simulink model "LW_ctrl"  (R2024b)
settings: Solver=ode4  StartTime=0.0  StopTime=SIM_TIME  FixedStep=0.001  RelTol=1e-3  EnableMultiTasking=on
StartFcn:
  | %timestart = cputime;
StopFcn:
  | %dt = cputime - timestart
undefined symbols (not defined in the file or in its folder): AttCtrl_cycle, ControlMode, DEG2RAD, Earth, FlightMode, LW_ACRO_P_MAX, LW_ACRO_R_MAX, LW_ACRO_Y_MAX, LW_AERO_C0, LW_AERO_C1, LW_AERO_Y0, LW_ANGLE, LW_DMZ0, LW_DMZ_MIN, LW_LAT_CIRCLE, LW_MAN_PITCH_MAX, LW_MAN_ROLL_MAX, LW_MASS, LW_OB_CIRCLE_R, LW_OB_CIRCLE_V, LW_OB_CIRCLE_W, LW_OB_TYPE, LW_REX_YAW, LW_SERVOL_MAX, LW_SERVOR_MAX, LW_THR_HOVER, LW_WZ_MAX, LW_X_ACCEL_MAX, LW_X_ACCEL_MIN, LW_X_FF, LW_X_JERK_MAX, LW_X_P, LW_X_VEL_MAX, LW_Y_ACCEL_MAX, LW_Y_ACCEL_MIN, LW_Y_FF, LW_Y_JERK_MAX, LW_Y_P, LW_Y_VEL_MAX, LW_YAW_KAD, LW_YAW_KAP, LW_Z_ACCEL_LOW, LW_Z_ACCEL_UP, LW_Z_FF, LW_Z_JERK_MAX, LW_Z_P, LW_Z_VEL_MAX_UP, Map_xoffset, Map_yoffset, Map_zoffset, MAX_wdotx, MAX_wdoty, MAX_wdotz, Mixer_cycle, ModelParam_AccelMax, ModelParam_DelayAtt, ModelParam_DelayOmega, ModelParam_DelayPos, ModelParam_envAltitude, ModelParam_envGravityAcc ... (+57)
libraries: pixhawk_slib_uORB_RW x15, simulink x6, slpidlib x6, dspstat3 x5, aerolibnav x4, aerolibtransform2 x3, pixhawk_slib_sensors_actuators x2, etargetslib x2, pixhawk_slib_rfly x1, aerolibatmos2 x1, slrealtimeiplib x1, SignalEditorBlockLib x1
(part 6 of 6)

== matlab function LW_ctrl/navigator/navigator_manual/vy_deadzone ==
  data: u input; y output; LW_Y_VEL_DZ parameter
function y = fcn(u, LW_Y_VEL_DZ)
%Function description:
%  set a dead zone with a dead zone size of ±deadZone.
RCMin = single(-1);
RCMax = single(1);
RCMid = ((RCMin + RCMax)/2);
deadZone = LW_Y_VEL_DZ;
k = 1/(RCMax - RCMid - deadZone);

%dead zone
if(u > RCMid + deadZone)
    y = single((u-RCMid - deadZone)*k);
elseif(u < RCMid - deadZone)
    y = single((u - RCMid + deadZone)*k);
else
    y = single(0);
end
end

== matlab function LW_ctrl/navigator/navigator_manual/vz_deadzone ==
  data: u input; y output; LW_Z_VEL_DZ parameter
function y = fcn(u, LW_Z_VEL_DZ)
%Function description:
%  set a dead zone with a dead zone size of ±deadZone.
% u:0-1
u = u*2 - 1; % -1~1
RCMin = single(-1);
RCMax = single(1);
RCMid = ((RCMin + RCMax)/2);
deadZone = LW_Z_VEL_DZ;
k = 1/(RCMax - RCMid - deadZone);

%dead zone
if(u > RCMid + deadZone)
    y = single((u-RCMid - deadZone)*k);
elseif(u < RCMid - deadZone)
    y = single((u - RCMid + deadZone)*k);
else
    y = single(0);
end
end

== matlab function LW_ctrl/rc_receive/manual_ctrl_in/Sim/Simulate ref/commandMapping/command2pwm/stabilized/roll_deadzone_inv ==
  data: u input; y output; LW_MAN_ROLL_DZ parameter
function y = fcn(u, LW_MAN_ROLL_DZ)
%Function description:
%  set a dead zone with a dead zone size of ±deadZone.
RCMin = single(-1);
RCMax = single(1);
RCMid = ((RCMin + RCMax)/2);
deadZone = LW_MAN_ROLL_DZ;
k = 1/(RCMax - RCMid - deadZone);

%dead zone
if(u > RCMid + deadZone)
    y = single(u/k + RCMid + deadZone);
elseif(u < RCMid - deadZone)
     y = single(u/k + RCMid - deadZone);
else
    y = single(0);
end
end

== matlab function LW_ctrl/rc_receive/manual_ctrl_in/Sim/Simulate ref/commandMapping/command2pwm/stabilized/pitch_deadzone_inv ==
  data: u input; y output; LW_MAN_PITCH_DZ parameter
function y = fcn(u, LW_MAN_PITCH_DZ)
%Function description:
%  set a dead zone with a dead zone size of ±deadZone.
RCMin = single(-1);
RCMax = single(1);
RCMid = ((RCMin + RCMax)/2);
deadZone = LW_MAN_PITCH_DZ;
k = 1/(RCMax - RCMid - deadZone);

%dead zone
if(u > RCMid + deadZone)
    y = single(u/k + RCMid + deadZone);
elseif(u < RCMid - deadZone)
     y = single(u/k + RCMid - deadZone);
else
    y = single(0);
end
end

== matlab function LW_ctrl/rc_receive/manual_ctrl_in/Sim/Simulate ref/commandMapping/command2pwm/stabilized/yawrare_deadzone_inv ==
  data: u input; y output; LW_MAN_WZ_DZ parameter
function y = fcn(u, LW_MAN_WZ_DZ)
%Function description:
%  set a dead zone with a dead zone size of ±deadZone.
RCMin = single(-1);
RCMax = single(1);
RCMid = ((RCMin + RCMax)/2);
deadZone = LW_MAN_WZ_DZ;
k = 1/(RCMax - RCMid - deadZone);

%dead zone
if(u > RCMid + deadZone)
    y = single(u/k + RCMid + deadZone);
elseif(u < RCMid - deadZone)
     y = single(u/k + RCMid - deadZone);
else
    y = single(0);
end
end

== matlab function LW_ctrl/rc_receive/manual_ctrl_in/Sim/Simulate ref/commandMapping/command2pwm/altitude/pitch_deadzone_inv ==
  data: u input; y output; LW_MAN_PITCH_DZ parameter
function y = fcn(u, LW_MAN_PITCH_DZ)
%Function description:
%  set a dead zone with a dead zone size of ±deadZone.
RCMin = single(-1);
RCMax = single(1);
RCMid = ((RCMin + RCMax)/2);
deadZone = LW_MAN_PITCH_DZ;
k = 1/(RCMax - RCMid - deadZone);

%dead zone
if(u > RCMid + deadZone)
    y = single(u/k + RCMid + deadZone);
elseif(u < RCMid - deadZone)
     y = single(u/k + RCMid - deadZone);
else
    y = single(0);
end
end

== matlab function LW_ctrl/rc_receive/manual_ctrl_in/Sim/Simulate ref/commandMapping/command2pwm/altitude/roll_deadzone_inv ==
  data: u input; y output; LW_MAN_ROLL_DZ parameter
function y = fcn(u, LW_MAN_ROLL_DZ)
%Function description:
%  set a dead zone with a dead zone size of ±deadZone.
RCMin = single(-1);
RCMax = single(1);
RCMid = ((RCMin + RCMax)/2);
deadZone = LW_MAN_ROLL_DZ;
k = 1/(RCMax - RCMid - deadZone);

%dead zone
if(u > RCMid + deadZone)
    y = single(u/k + RCMid + deadZone);
elseif(u < RCMid - deadZone)
     y = single(u/k + RCMid - deadZone);
else
    y = single(0);
end
end

== matlab function LW_ctrl/rc_receive/manual_ctrl_in/Sim/Simulate ref/commandMapping/command2pwm/acro/wz_deadzone_inv ==
  data: u input; y output; LW_MAN_WZ_DZ parameter
function y = fcn(u, LW_MAN_WZ_DZ)
%Function description:
%  set a dead zone with a dead zone size of ±deadZone.
RCMin = single(-1);
RCMax = single(1);
RCMid = ((RCMin + RCMax)/2);
deadZone = LW_MAN_WZ_DZ;
k = 1/(RCMax - RCMid - deadZone);

%dead zone
if(u > RCMid + deadZone)
    y = single(u/k + RCMid + deadZone);
elseif(u < RCMid - deadZone)
     y = single(u/k + RCMid - deadZone);
else
    y = single(0);
end
end

== matlab function LW_ctrl/rc_receive/manual_ctrl_in/Sim/Simulate ref/commandMapping/command2pwm/acro/wx_deadzone_inv ==
  data: u input; y output; LW_MAN_WX_DZ parameter
function y = fcn(u, LW_MAN_WX_DZ)
%Function description:
%  set a dead zone with a dead zone size of ±deadZone.
RCMin = single(-1);
RCMax = single(1);
RCMid = ((RCMin + RCMax)/2);
deadZone = LW_MAN_WX_DZ;
k = 1/(RCMax - RCMid - deadZone);

%dead zone
if(u > RCMid + deadZone)
    y = single(u/k + RCMid + deadZone);
elseif(u < RCMid - deadZone)
     y = single(u/k + RCMid - deadZone);
else
    y = single(0);
end
end

== matlab function LW_ctrl/rc_receive/manual_ctrl_in/Sim/Simulate ref/commandMapping/command2pwm/acro/wy_deadzone_inv ==
  data: u input; y output; LW_MAN_WY_DZ parameter
function y = fcn(u, LW_MAN_WY_DZ)
%Function description:
%  set a dead zone with a dead zone size of ±deadZone.
RCMin = single(-1);
RCMax = single(1);
RCMid = ((RCMin + RCMax)/2);
deadZone = LW_MAN_WY_DZ;
k = 1/(RCMax - RCMid - deadZone);

%dead zone
if(u > RCMid + deadZone)
    y = single(u/k + RCMid + deadZone);
elseif(u < RCMid - deadZone)
     y = single(u/k + RCMid - deadZone);
else
    y = single(0);
end
end

== matlab function LW_ctrl/rc_receive/manual_ctrl_in/Sim/Simulate ref/commandMapping/command2pwm/position/wz_deadzone_inv ==
  data: u input; y output; LW_MAN_WZ_DZ parameter
function y = fcn(u, LW_MAN_WZ_DZ)
%Function description:
%  set a dead zone with a dead zone size of ±deadZone.
RCMin = single(-1);
RCMax = single(1);
RCMid = ((RCMin + RCMax)/2);
deadZone = LW_MAN_WZ_DZ;
k = 1/(RCMax - RCMid - deadZone);

%dead zone
if(u > RCMid + deadZone)
    y = single(u/k + RCMid + deadZone);
elseif(u < RCMid - deadZone)
     y = single(u/k + RCMid - deadZone);
else
    y = single(0);
end
end

== matlab function LW_ctrl/rc_receive/manual_ctrl_in/Sim/Simulate ref/commandMapping/command2pwm/position/vz_deadzone_inv ==
  data: u input; y output; LW_Z_VEL_DZ parameter
function y = fcn(u, LW_Z_VEL_DZ)
%Function description:
%  set a dead zone with a dead zone size of ±deadZone.
RCMin = single(-1);
RCMax = single(1);
RCMid = ((RCMin + RCMax)/2);
deadZone = LW_Z_VEL_DZ;
k = 1/(RCMax - RCMid - deadZone);

%dead zone
if(u > RCMid + deadZone)
    y = single(u/k + RCMid + deadZone);
elseif(u < RCMid - deadZone)
     y = single(u/k + RCMid - deadZone);
else
    y = single(0);
end

y = (y+1)*0.5;
end

== matlab function LW_ctrl/rc_receive/manual_ctrl_in/Sim/Simulate ref/commandMapping/command2pwm/position/vy_deadzone_inv ==
  data: u input; y output; LW_Y_VEL_DZ parameter
function y = fcn(u, LW_Y_VEL_DZ)
%Function description:
%  set a dead zone with a dead zone size of ±deadZone.
RCMin = single(-1);
RCMax = single(1);
RCMid = ((RCMin + RCMax)/2);
deadZone = LW_Y_VEL_DZ;
k = 1/(RCMax - RCMid - deadZone);

%dead zone
if(u > RCMid + deadZone)
    y = single(u/k + RCMid + deadZone);
elseif(u < RCMid - deadZone)
     y = single(u/k + RCMid - deadZone);
else
    y = single(0);
end
end

== matlab function LW_ctrl/rc_receive/manual_ctrl_in/Sim/Simulate ref/commandMapping/command2pwm/position/vx_deadzone_inv ==
  data: u input; y output; LW_X_VEL_DZ parameter
function y = fcn(u, LW_X_VEL_DZ)
%Function description:
%  set a dead zone with a dead zone size of ±deadZone.
RCMin = single(-1);
RCMax = single(1);
RCMid = ((RCMin + RCMax)/2);
deadZone = LW_X_VEL_DZ;
k = 1/(RCMax - RCMid - deadZone);

%dead zone
if(u > RCMid + deadZone)
    y = single(u/k + RCMid + deadZone);
elseif(u < RCMid - deadZone)
     y = single(u/k + RCMid - deadZone);
else
    y = single(0);
end
end

== matlab function LW_ctrl/rc_receive/manual_ctrl_in/Sim/Simulate ref/commandMapping/command2pwm/altitude/vz_deadzone_inv ==
  data: u input; y output; LW_Z_VEL_DZ parameter
function y = fcn(u, LW_Z_VEL_DZ)
%Function description:
%  set a dead zone with a dead zone size of ±deadZone.
RCMin = single(-1);
RCMax = single(1);
RCMid = ((RCMin + RCMax)/2);
deadZone = LW_Z_VEL_DZ;
k = 1/(RCMax - RCMid - deadZone);

%dead zone
if(u > RCMid + deadZone)
    y = single(u/k + RCMid + deadZone);
elseif(u < RCMid - deadZone)
     y = single(u/k + RCMid - deadZone);
else
    y = single(0);
end

y = (y+1)*0.5;
end

== matlab function LW_ctrl/rc_receive/manual_ctrl_in/Sim/Simulate ref/commandMapping/command2pwm/altitude/wz_deadzone_inv ==
  data: u input; y output; LW_MAN_WZ_DZ parameter
function y = fcn(u, LW_MAN_WZ_DZ)
%Function description:
%  set a dead zone with a dead zone size of ±deadZone.
RCMin = single(-1);
RCMax = single(1);
RCMid = ((RCMin + RCMax)/2);
deadZone = LW_MAN_WZ_DZ;
k = 1/(RCMax - RCMid - deadZone);

%dead zone
if(u > RCMid + deadZone)
    y = single(u/k + RCMid + deadZone);
elseif(u < RCMid - deadZone)
     y = single(u/k + RCMid - deadZone);
else
    y = single(0);
end
end

== matlab function LW_ctrl/states_update/vehicle_local_position/Sim/getIncid ==
  data: q input; incid output; LW_ANGLE parameter
function incid = fcn(q, LW_ANGLE)

if notInfNan(q)
    euler = my_quat2eul(q);
else
    euler = single([0;0;0]);
end
theta = euler(2);
alpha = theta + LW_ANGLE*pi/180;
beta = single(0);
incid = [alpha; beta];

== matlab function LW_ctrl/navigator/navigator_manual/Lowpass ==
  data: data_in input; data_in output; LW_VEL_DT parameter
function data_in = fcn(data_in, LW_VEL_DT)
persistent data_last
if isempty(data_last)
    data_last = data_in;
end
if isInfNan(data_last)
    data_last = single(0);
end

data_in = data_last + LW_VEL_DT*(data_in - data_last);
data_last = data_in;

== matlab function LW_ctrl/navigator/navigator_manual/Lowpass1 ==
  data: data_in input; data_in output; LW_VEL_DT parameter
function data_in = fcn(data_in, LW_VEL_DT)
persistent data_last
if isempty(data_last)
    data_last = data_in;
end
if isInfNan(data_last)
    data_last = single(0);
end

data_in = data_last + LW_VEL_DT*(data_in - data_last);
data_last = data_in;

== matlab function LW_ctrl/Output/OutputSelect/Sim/Lifting Body Airframe/Estimator/Sensor Model/GPS/GenCogVel ==
  data: v output; u input; cot output
function [v,cot] = Ang360(u)
v=norm(u(1:2));

if v < 1
    cot = 0;
else
    cot=atan2d(u(2),u(1));
end
 
if cot<0
    cot=cot+360;
end

== matlab function LW_ctrl/navigator/logger/Sim/quat2eul ==
  data: q input; euler output
function euler = fcn(q)
q = single(q);
euler = my_quat2eul(q,'ZYX');

== matlab function LW_ctrl/Output/OutputSelect/Sim/Lifting Body Airframe/Estimator/Sensor Model/Magnetometer Hub/MATLAB Function ==
  data: DCM input; mag_e input; b_m input; n_m input; Mag_means output; K_m input
function Mag_means = fcn(DCM, mag_e, b_m, n_m, K_m)
 
Mag_means = K_m*DCM*mag_e + b_m + n_m;

== matlab function LW_ctrl/Output/OutputSelect/Sim/Lifting Body Airframe/Estimator/Sensor Model/Magnetometer Hub/MATLAB Function1 ==
  data: DCM input; mag_e input; b_m input; n_m input; Mag_means output; K_m input
function Mag_means = fcn(DCM, mag_e, b_m, n_m, K_m)
 
Mag_means = K_m*DCM*mag_e + b_m + n_m;

== matlab function LW_ctrl/navigator/navigator_manual/nan_inf0 ==
  data: u input; y output
function y = fcn(u)

for i = 1:length(u)
    if isnan(u(i)) || isinf(u(i))
        u(i) = single(0);
    end
end
y = u;

== matlab function LW_ctrl/navigator/navigator_manual/nan_inf1 ==
  data: u input; y output
function y = fcn(u)

for i = 1:length(u)
    if isnan(u(i)) || isinf(u(i))
        u(i) = single(0);
    end
end
y = u;

== matlab function LW_ctrl/navigator/navigator_manual/nan_inf2 ==
  data: u input; y output
function y = fcn(u)

for i = 1:length(u)
    if isnan(u(i)) || isinf(u(i))
        u(i) = single(0);
    end
end
y = u;

== matlab function LW_ctrl/navigator/navigator_manual/nan_inf3 ==
  data: u input; y output
function y = fcn(u)

for i = 1:length(u)
    if isnan(u(i)) || isinf(u(i))
        u(i) = single(0);
    end
end
y = u;

== matlab function LW_ctrl/navigator/navigator_manual/nan_inf4 ==
  data: u input; y output
function y = fcn(u)

for i = 1:length(u)
    if isnan(u(i)) || isinf(u(i))
        u(i) = single(0);
    end
end
y = u;

== matlab function LW_ctrl/navigator/navigator_manual/nan_inf5 ==
  data: u input; y output
function y = fcn(u)

for i = 1:length(u)
    if isnan(u(i)) || isinf(u(i))
        u(i) = single(0);
    end
end
y = u;

== matlab function LW_ctrl/navigator/navigator_manual/nan_inf6 ==
  data: u input; y output
function y = fcn(u)

for i = 1:length(u)
    if isnan(u(i)) || isinf(u(i))
        u(i) = single(0);
    end
end
y = u;

== matlab function LW_ctrl/navigator/navigator_manual/nan_inf7 ==
  data: u input; y output
function y = fcn(u)

for i = 1:length(u)
    if isnan(u(i)) || isinf(u(i))
        u(i) = single(0);
    end
end
y = u;

== matlab function LW_ctrl/navigator/navigator_manual/nan_inf8 ==
  data: u input; y output
function y = fcn(u)

for i = 1:length(u)
    if isnan(u(i)) || isinf(u(i))
        u(i) = single(0);
    end
end
y = u;

== matlab function LW_ctrl/rc_receive/manual_ctrl_in/Sim/Simulate ref/commandMapping/MATLAB Function ==
  data: flight_mode input; AU8 output
function AU8 = fcn(flight_mode)
if flight_mode == FlightMode.PILOT
    AU8 = 1000;
elseif flight_mode == FlightMode.AUTO
    AU8 = 1500;
else
    %offboard
    AU8 = 2000;
end

== matlab function LW_ctrl/state_machine/MATLAB Function4 ==
  data: ctrl_mode output; ch5 input; ch7 input; ch8 input; flight_mode output; RC_Lost input; armed input
function [ctrl_mode, flight_mode]  = fcn(ch5, ch7, ch8, RC_Lost, armed)
%Function description:
%  Map the remote control CH5 channel to control mode
%input:
%  ch5: Remote control CH5 channel input
%  control_mode: Custom control mode
%  0: stablelize mode；1: height control mode; 2: position control mode
%  4: attitude rate mode
%  the remote control CH8 channel change the flight mode
%input:
%  ch8: Remote control CH8 channel input

if ch5 < 1400
    ctrl_mode = ControlMode.STABILIZED;
    if ch7 >1300 && ch7 < 1600
        %ctrl_mode = ControlMode.ACRO;
    elseif ch7 >= 1600
        ctrl_mode = ControlMode.MANUAL;
    end
elseif ch5 < 1600
    ctrl_mode = ControlMode.ALTITUDE;
else
    ctrl_mode = ControlMode.POSITION;
end
if ch8 < 1400
    flight_mode = FlightMode.PILOT;
% elseif ch8 < 1600
%     flight_mode = FlightMode.AUTO;
%     ctrl_mode = ControlMode.MISSION;
else
    flight_mode = FlightMode.OFFBOARD;
end

if RC_Lost > 0.5
%     flight_mode = FlightMode.AUTO;
%     ctrl_mode = ControlMode.LOITER;
end

% if armed > 0.5 && ch8 > 1500
%     flight_mode = FlightMode.OFFBOARD;
% end

== matlab function LW_ctrl/Output/OutputSelect/Sim/Lifting Body Airframe/Estimator/nan_inf ==
  data: u input; y output
function y = fcn(u)

for i = 1:length(u)
    if isnan(u(i)) || isinf(u(i))
        u(i) = 0;
    end
end
y = u;

== matlab function LW_ctrl/Output/OutputSelect/Sim/Lifting Body Airframe/Estimator/nan_inf1 ==
  data: u input; y output
function y = fcn(u)

for i = 1:length(u)
    if isnan(u(i)) || isinf(u(i))
        u(i) = 0;
    end
end
y = u;

== matlab function LW_ctrl/navigator/navigator_manual/nan_inf10 ==
  data: u input; y output
function y = fcn(u)

for i = 1:length(u)
    if isnan(u(i)) || isinf(u(i))
        u(i) = single(0);
    end
end
y = u;

== matlab function LW_ctrl/Output/OutputSelect/Sim/Lifting Body Airframe/Estimator/nan_inf2 ==
  data: u input; y output
function y = fcn(u)

for i = 1:length(u)
    if isnan(u(i)) || isinf(u(i))
        u(i) = 0;
    end
end
y = u;

== matlab function LW_ctrl/Output/OutputSelect/Sim/Lifting Body Airframe/Estimator/nan_inf3 ==
  data: u input; y output
function y = fcn(u)

for i = 1:length(u)
    if isnan(u(i)) || isinf(u(i))
        u(i) = 0;
    end
end
y = u;

== matlab function LW_ctrl/Output/OutputSelect/Sim/Lifting Body Airframe/Estimator/nan_inf4 ==
  data: u input; y output
function y = fcn(u)

for i = 1:length(u)
    if isnan(u(i)) || isinf(u(i))
        u(i) = 0;
    end
end
y = u;

== matlab function LW_ctrl/Output/OutputSelect/Sim/Lifting Body Airframe/Estimator/nan_inf5 ==
  data: u input; y output
function y = fcn(u)

for i = 1:length(u)
    if isnan(u(i)) || isinf(u(i))
        u(i) = 0;
    end
end
y = u;

== matlab function LW_ctrl/Output/OutputSelect/Sim/Lifting Body Airframe/Estimator/nan_inf6 ==
  data: u input; y output
function y = fcn(u)

for i = 1:length(u)
    if isnan(u(i)) || isinf(u(i))
        u(i) = 15;
    end
end
y = u;

== matlab function LW_ctrl/Output/OutputSelect/Sim/Lifting Body Airframe/Estimator/nan_inf_q ==
  data: u input; y output
function y = fcn(u)

for i = 1:length(u)
    if isnan(u(i)) || isinf(u(i))
        if i == 1
            u(i) = 1;
        else
            u(i) = 0;
        end
    end
end
y = u;

== matlab function LW_ctrl/Output/OutputSelect/Sim/Lifting Body Airframe/Get Terrain/getTerrainAltData ==
  settings: updateMethod=DISCRETE
  data: x input; z output; y input
function z = fcn(x,y)
%z=getTerrainAltData(x,y);
persistent zoffset
if isnan(x) || isnan(y)
   x = 0;
   y = 0;
end
if isempty(zoffset)
    zoffset = getTerrainAltData(x,y);
end
z=getTerrainAltData(x,y) - zoffset;

end

== matlab function LW_ctrl/navigator/navigator_manual/Lowpass2 ==
  data: data_in input; data_in output; LW_VEL_DT parameter
function data_in = fcn(data_in, LW_VEL_DT)
persistent data_last
if isempty(data_last)
    data_last = data_in;
end
if isInfNan(data_last)
    data_last = single(0);
end

data_in = data_last + LW_VEL_DT*(data_in - data_last);
data_last = data_in;

== matlab function LW_ctrl/navigator/navigator_offboard/task select/task select/task ==
  data: timestamp input; flight_mode input; pos input size=[3,1]; vel input size=[3,1]; q input; pos_ref output size=[3,1]; vel_ref output size=[3,1]; acc_ref output; euler_ref output; dot3x output; yaw_ref output; dotpsi output; LW_OB_CIRCLE_R parameter; LW_OB_CIRCLE_V parameter; LW_OB_CIRCLE_W parameter; LW_OB_TYPE parameter; reverse_flag output; CH8 input
function [pos_ref, vel_ref, acc_ref, euler_ref,dot3x, yaw_ref, dotpsi,reverse_flag] = fcn(timestamp, flight_mode,pos, vel, q, LW_OB_CIRCLE_R, LW_OB_CIRCLE_V, LW_OB_CIRCLE_W, LW_OB_TYPE,CH8)

if CH8 < 1600
    [pos_ref, vel_ref, acc_ref, euler_ref,dot3x, yaw_ref, dotpsi,reverse_flag] = task5(timestamp, flight_mode,pos, vel, q, LW_OB_CIRCLE_R, LW_OB_CIRCLE_V, LW_OB_CIRCLE_W, LW_OB_TYPE);
else
    [pos_ref, vel_ref, acc_ref, euler_ref,dot3x, yaw_ref, dotpsi,reverse_flag] = task1(timestamp, flight_mode,pos, vel, q, LW_OB_CIRCLE_R, LW_OB_CIRCLE_V, LW_OB_CIRCLE_W, LW_OB_TYPE);
end
end

== matlab function LW_ctrl/navigator/navigator_offboard/task select/task select/df,coor,wind ==
  data: pos_ref input; vel_ref input; acc_ref input; euler_ref input; dot3x input; yaw_ref input; dotpsi input; v_wind input; pos_ref output; vel_ref output; acc_ref output; q_ref output; f_d output; alpha output; beta output; wb_ref output; dotwb_ref output; ModelParam_LBRho parameter; ModelParam_LBS parameter; ModelParam_pu_c0 parameter; ModelParam_pu_c1 parameter; LW_AERO_Y0 parameter; LW_ANGLE parameter; ModelParam_pu_c2 parameter; ModelParam_pu_c3 parameter; ModelParam_envGravityAcc parameter; LW_AERO_C0 parameter; LW_AERO_C1 parameter; LW_MASS parameter; OB_TASK output; eee output
function [pos_ref, vel_ref, acc_ref, q_ref, f_d, alpha,beta, wb_ref, dotwb_ref, OB_TASK,eee] = fcn(pos_ref, vel_ref, acc_ref, euler_ref, dot3x, yaw_ref, dotpsi, v_wind, ...
    ModelParam_LBRho, ModelParam_LBS, ModelParam_pu_c0, ModelParam_pu_c1, LW_AERO_Y0, LW_ANGLE, ModelParam_pu_c2, ModelParam_pu_c3, ModelParam_envGravityAcc, LW_AERO_C0, LW_AERO_C1, LW_MASS)

% Note
% adopt the results from differential Flatness derived from data 2022-6-16
% 加入风

persistent xw_  yb_
if isempty(xw_)
    if ~isnan(yaw_ref)
        xw_ = [cos(yaw_ref) sin(yaw_ref) 0]';
        yb_ = [-sin(yaw_ref) cos(yaw_ref) 0]';
    else
        xw_ = single([1 0 0]');
        yb_ = single([0 1 0]');
    end 
end
%% 
airspeed_T = single(0.01);
g = single([0; 0; ModelParam_envGravityAcc]);
Cd0 = single(ModelParam_pu_c0); % 最小阻力
Cla = single(ModelParam_pu_c1); % post stall
Cd0 = single(LW_AERO_C0); % 最小阻力
Cla = single(LW_AERO_C1); % post stall

% Cd0 = single(ModelParam_pu_c3); % 最小阻力
% Cla = single(ModelParam_pu_c2); % pre stall
Cy0 = single(LW_AERO_Y0);
kk = single(LW_ANGLE*pi/180);
Rho = single(ModelParam_LBRho);
Mass = single(LW_MASS);


dotdotx = single(acc_ref(:));
va = single(vel_ref(:) - v_wind);
Va = sqrt(va'*va);
Qa = 0.5/Mass * Rho * ModelParam_LBS * Va;

if ~isnan(yaw_ref)
    xw_ = [cos(yaw_ref) sin(yaw_ref) 0]';
    yb_ = [-sin(yaw_ref) cos(yaw_ref) 0]';
end

if Va > airspeed_T && isnan(yaw_ref)
    xw = va / Va;
    xw_ = xw;
else
    xw = xw_;
end

    a_xw = xw' * (dotdotx - g);
    an = dotdotx - g - a_xw * xw;
    a_zw = -norm(an);
    [f_d, alpha] = SolveFza(a_xw, a_zw, Va, Cd0, Cla, Rho,  ModelParam_LBS, LW_MASS, kk);

    ay = Qa * Cy0 * va - g + dotdotx;
    xw_ay_norm = norm(cross(xw, ay));
    if xw_ay_norm > 0.01
        yb = cross(xw, ay) / xw_ay_norm;
        yb_ = yb;
    else
        yb = yb_;
    end
    yb_hat = [0 -yb(3) yb(2); yb(3) 0 -yb(1); -yb(2) yb(1) 0];
    lamda = alpha - kk;
    xb = (cos(lamda)*eye(3) + (1 - cos(lamda))*yb*yb'+sin(lamda)*yb_hat)*xw;
    zb = cross(xb, yb);
    R_d = [xb yb zb];
    %协调假设求解角速度
    wb_ref = calculateWb(f_d, R_d, Va, va, dotdotx, dot3x, Cd0, Cla, Cy0, Rho, ModelParam_LBS, LW_MASS, g, kk);
    q_ref = R2quat(R_d);
    dotwb_ref = zeros(3,1,'single');
    beta = single(0);
    OB_TASK = int8(2);
    eee = my_quat2eul(q_ref);
end

function [fz, alpha] = SolveFza(av1_, av3_, Va, Cd0, Cla, Rho, S, m, kk)

Q = 0.5 * Rho * Va ^ 2;
QSCla = Q * S * Cla;

av1 = av1_*m + Q * S * Cd0;
av3 = min(av3_*m, 0);
k1 = sqrt(av1 ^ 2 * cos(kk) ^ 2 + (av1 + QSCla) ^ 2 * sin(kk) ^ 2 + av3 ^ 2 - QSCla * av3 * sin(2 * kk));
fz = -(av1^2 + QSCla*av1 + av3^2) / k1;

alpha = 2 * atan((QSCla * sin(kk) - av3 * cos(kk) + av1 * sin(kk) - k1) / (av1 * cos(kk) + av3 * sin(kk)));
end

function wbb = calculateWb(fz, Rbb, Vg, dotx, dotdotx, dot3x, Cd0, Cla, Cy0, Rho, S, m, g, kk)
    persistent wz_ wx_
    if isempty(wz_)
        wz_ = single(0);
        wx_ = single(0);
    end
    Qa = 0.5/m * Rho * S * Vg;
    cz = fz/m;
    dxz = Cla * sin(kk) * cos(kk);
    dx = Cd0 + Cla * sin(kk) ^ 2;
    dz = Cd0 + Cla * cos(kk) ^ 2;
    
    if Vg < 0.01
        C1 = Rbb(:, 1)' * dot3x + Qa * (dx * Rbb(:, 1)' * dotdotx + dxz * Rbb(:, 3)' * dotdotx);
    else
        C1 = Rbb(:, 1)' * dot3x + Qa*dotx'*dotdotx/(Vg^2)*(dx * Rbb(:, 1)' * dotx + dxz * Rbb(:, 3)' * dotx)+ Qa * (dx * Rbb(:, 1)' * dotdotx + dxz * Rbb(:, 3)' * dotdotx);
    end
    
    A1 = Qa * dxz * Rbb(:, 2)' * dotx;
    B1 = cz - Qa * ((dz - dx) * Rbb(:, 3)' * dotx + 2*dxz * Rbb(:, 1)' * dotx);
    D1 = -Qa * ((dx - Cy0) * Rbb(:, 2)' * dotx);
    if Vg < 0.01
        C2 = Rbb(:, 2)' * dot3x + Qa * Cy0 * Rbb(:, 2)' * dotdotx;
    else
        C2 = Rbb(:, 2)' * dot3x + Qa*dotx'*dotdotx/(Vg^2)*(Cy0 * Rbb(:, 2)' * dotx)+ Qa * Cy0 * Rbb(:, 2)' * dotdotx;
    end
    A2 = -cz + Qa * (dxz * Rbb(:, 1)' * dotx + (dz - Cy0) * Rbb(:, 3)' * dotx);
    D2 = -Qa * ((dx - Cy0) * Rbb(:, 1)' * dotx + dxz * Rbb(:, 3)' * dotx);
    A3 = Rbb(:, 3)' * dotx;
    D3 = -Rbb(:, 1)' * dotx;
    C3 = -Rbb(:, 2)' * g;
    if abs(A2*D3 - A3*D2) < 0.001
        wz = wz_;
        wx = (C2 - D2*wz)/A2;
        %wx = wx_;
        wy = (C1 - A1*wx - D1*wz)/B1;
        %disp('Omega Signarity')
    else
        wx = (C2*D3 - C3*D2)/(A2*D3 - A3*D2);
        wy = -(A1*C2*D3 - A1*C3*D2 - A2*C1*D3 + A2*C3*D1 + A3*C1*D2 - A3*C2*D1)/(B1*(A2*D3 - A3*D2));
        wz = (A2*C3 - A3*C2)/(A2*D3 - A3*D2);
        wz_ = wz;
        wx_ = wx;
    end
%     wx = -(D2*wsz - C2*cos(kk-alpha))/(A2*cos(kk-alpha) + D2*sin(kk-alpha));
%     wy = (A1*D2*wsz - A2*D1*wsz - A1*C2*cos(kk-alpha) + A2*C1*cos(kk-alpha) + C1*D2*sin(kk-alpha) - C2*D1*sin(kk-alpha))/(B1*(A2*cos(kk-alpha) + D2*sin(kk-alpha)));
%     wz = (A2*wsz + C2*sin(kk-alpha))/(A2*cos(kk-alpha) + D2*sin(kk-alpha));
    wbb = [wx; wy; wz];
    %wbb(2) = constrain(wbb(2), -3, 3); wbb(1) = constrain(wbb(1), -3, 3); wbb(3) = constrain(wbb(3), -3, 3);
end

== matlab function LW_ctrl/Output/OutputSelect/HIL/MATLAB Function2 ==
  data: LW_LED parameter; LW_USE_SER parameter; LW_COOR_TURN parameter; LW_AERO_COM parameter; LW_TEST_EN parameter; LW_FEST_EN parameter; LW_F_MAP parameter; LW_REX_YAW parameter; LW_DMZ0 parameter; LW_DMZ_MIN parameter; LW_YAW_KAP parameter; LW_YAW_KAD parameter; LW_ANGLE parameter; LW_MASS parameter; LW_THR_HOVER parameter; LW_THR_LOW parameter; LW_DTHR parameter; LW_DSER parameter; LW_AERO_C0 parameter; LW_AERO_C1 parameter; LW_AERO_Y0 parameter; LW_LBCL_D parameter; LW_LBCM_D parameter; LW_OB_TYPE parameter; LW_FEST_WNXY parameter; LW_FEST_WNZ parameter; LW_FEST_SIGXY parameter; LW_FEST_SIGZ parameter; LW_FEST_LAMXY parameter; LW_FEST_LAMZ parameter; LW_FEST_P parameter; LW_FEST_DT parameter; LW_FEST_TDT parameter; LW_TEST_WNXY parameter; LW_TEST_WNZ parameter; LW_TEST_SIGXY parameter; LW_TEST_SIGZ parameter; LW_TEST_LAMXY parameter; LW_TEST_LAMZ parameter; LW_TEST_DTXY parameter; LW_TEST_DTZ parameter; LW_TEST_WBDT parameter; LW_TEST_TDT parameter; LW_VA_TMIN parameter; LW_VA_TMAX parameter; LW_MIXER_GAM parameter; LW_W_FZ parameter; LW_W_TAOX parameter; LW_W_TAOY parameter; LW_W_TAOZ parameter; LW_W_SER parameter; LW_W_SERH parameter; LW_SER_LP parameter; LW_MAN_ROLL_MAX parameter; LW_MAN_PITCH_MAX parameter; LW_WY_MAX parameter; LW_WY_DE_MAX parameter; LW_WX_MAX parameter; LW_WZ_MAX parameter; LW_ACRO_P_MAX parameter; LW_ACRO_R_MAX parameter; LW_ACRO_Y_MAX parameter; LW_PITCH_P parameter; LW_WY_P parameter; LW_WY_I parameter; LW_WY_D parameter; LW_WY_N parameter; LW_ROLL_P parameter; LW_WX_P parameter; LW_WX_I parameter; LW_WX_D parameter; LW_WX_N parameter; LW_YAW_P parameter; LW_WZ_P parameter; LW_WZ_I parameter; LW_WZ_D parameter; LW_WZ_N parameter; LW_WX_FF parameter; LW_WY_FF parameter; LW_WZ_FF parameter; LW_TAUXYSP_FZ parameter; LW_TAUXYSP_TM parameter; LW_TAUZSP_FZ parameter; LW_TAUZSP_TM parameter; LW_ACCSP_FZ parameter; LW_ACCSP_TM parameter; LW_TILTMAX_AIR parameter; LW_LAT_CIRCLE parameter; LW_X_VEL_MAX parameter; LW_X_ACCEL_MAX parameter; LW_X_ACCEL_MIN parameter; LW_X_JERK_MAX parameter; LW_Y_VEL_MAX parameter; LW_Y_ACCEL_MAX parameter; LW_Y_ACCEL_MIN parameter; LW_Y_JERK_MAX parameter; LW_Z_VEL_MAX_UP parameter; LW_Z_ACCEL_LOW parameter; LW_Z_ACCEL_UP parameter; LW_Z_JERK_MAX parameter; LW_VEL_DT parameter; LW_X_FF parameter; LW_Y_FF parameter; LW_Z_FF parameter; LW_X_P parameter; LW_X_VEL_P parameter; LW_X_VEL_I parameter; LW_X_VEL_D parameter; LW_X_VEL_N parameter; LW_Y_P parameter; LW_Y_VEL_P parameter; LW_Y_VEL_I parameter; LW_Y_VEL_D parameter; LW_Y_VEL_N parameter; LW_Z_P parameter; LW_Z_VEL_P parameter; LW_Z_VEL_I parameter; LW_Z_VEL_D parameter; LW_Z_VEL_N parameter; LW_ACCX_FF parameter; LW_ACCY_FF parameter; LW_ACCZ_FF parameter; LW_OB_CIRCLE_R parameter; LW_OB_CIRCLE_V parameter; LW_OB_CIRCLE_W parameter; RC1_MIN parameter; RC1_MAX parameter; RC1_REV parameter; RC2_MIN parameter; RC2_MAX parameter; RC2_REV parameter; RC3_MIN parameter; RC3_MAX parameter; RC3_REV parameter; RC4_MIN parameter; RC4_MAX parameter; RC4_REV parameter; LW_MAN_ROLL_DZ parameter; LW_MAN_PITCH_DZ parameter; LW_MAN_WX_DZ parameter; LW_MAN_WY_DZ parameter; LW_MAN_WZ_DZ parameter; LW_X_VEL_DZ parameter; LW_Y_VEL_DZ parameter; LW_Z_VEL_DZ parameter; LW_SERVOR_REV parameter; LW_SERVOL_REV parameter; LW_SERVOR_MAX parameter; LW_SERVOR_MIN parameter; LW_SERVOL_MAX parameter; LW_SERVOL_MIN parameter; LW_SERVOR_CON parameter; out output
function out  = yourFcn( ...
LW_LED, LW_USE_SER, LW_COOR_TURN, LW_AERO_COM, LW_TEST_EN, LW_FEST_EN, LW_F_MAP, LW_REX_YAW, ...
LW_DMZ0, LW_DMZ_MIN, LW_YAW_KAP, LW_YAW_KAD, LW_ANGLE, ...
LW_MASS, LW_THR_HOVER, LW_THR_LOW, LW_DTHR, LW_DSER, LW_AERO_C0, LW_AERO_C1, LW_AERO_Y0, LW_LBCL_D, LW_LBCM_D, LW_OB_TYPE, ...
LW_FEST_WNXY, LW_FEST_WNZ, LW_FEST_SIGXY, LW_FEST_SIGZ, LW_FEST_LAMXY, LW_FEST_LAMZ, LW_FEST_P, LW_FEST_DT, LW_FEST_TDT, ...
LW_TEST_WNXY, LW_TEST_WNZ, LW_TEST_SIGXY, LW_TEST_SIGZ, LW_TEST_LAMXY, LW_TEST_LAMZ, LW_TEST_DTXY, LW_TEST_DTZ, LW_TEST_WBDT, LW_TEST_TDT, ...
LW_VA_TMIN, LW_VA_TMAX, LW_MIXER_GAM, LW_W_FZ, LW_W_TAOX, LW_W_TAOY, LW_W_TAOZ, LW_W_SER, LW_W_SERH, LW_SER_LP, ...
LW_MAN_ROLL_MAX, LW_MAN_PITCH_MAX, LW_WY_MAX, LW_WY_DE_MAX, LW_WX_MAX, LW_WZ_MAX, LW_ACRO_P_MAX, LW_ACRO_R_MAX, LW_ACRO_Y_MAX, ...
LW_PITCH_P, LW_WY_P, LW_WY_I, LW_WY_D, LW_WY_N, LW_ROLL_P, LW_WX_P, LW_WX_I, LW_WX_D, LW_WX_N, LW_YAW_P, LW_WZ_P, LW_WZ_I, LW_WZ_D, LW_WZ_N, ...
LW_WX_FF, LW_WY_FF, LW_WZ_FF, LW_TAUXYSP_FZ, LW_TAUXYSP_TM, LW_TAUZSP_FZ, LW_TAUZSP_TM, LW_ACCSP_FZ, LW_ACCSP_TM, ...
LW_TILTMAX_AIR, LW_LAT_CIRCLE, LW_X_VEL_MAX, LW_X_ACCEL_MAX, LW_X_ACCEL_MIN, LW_X_JERK_MAX, LW_Y_VEL_MAX, LW_Y_ACCEL_MAX, LW_Y_ACCEL_MIN, LW_Y_JERK_MAX, ...
LW_Z_VEL_MAX_UP, LW_Z_ACCEL_LOW, LW_Z_ACCEL_UP, LW_Z_JERK_MAX, LW_VEL_DT, ...
LW_X_FF, LW_Y_FF, LW_Z_FF, LW_X_P, LW_X_VEL_P, LW_X_VEL_I, LW_X_VEL_D, LW_X_VEL_N, LW_Y_P, LW_Y_VEL_P, LW_Y_VEL_I, LW_Y_VEL_D, LW_Y_VEL_N, ...
LW_Z_P, LW_Z_VEL_P, LW_Z_VEL_I, LW_Z_VEL_D, LW_Z_VEL_N, LW_ACCX_FF, LW_ACCY_FF, LW_ACCZ_FF, ...
LW_OB_CIRCLE_R, LW_OB_CIRCLE_V, LW_OB_CIRCLE_W, ...
RC1_MIN, RC1_MAX, RC1_REV, RC2_MIN, RC2_MAX, RC2_REV, RC3_MIN, RC3_MAX, RC3_REV, RC4_MIN, RC4_MAX, RC4_REV, ...
LW_MAN_ROLL_DZ, LW_MAN_PITCH_DZ, LW_MAN_WX_DZ, LW_MAN_WY_DZ, LW_MAN_WZ_DZ, LW_X_VEL_DZ, LW_Y_VEL_DZ, LW_Z_VEL_DZ, ...
LW_SERVOR_REV, LW_SERVOL_REV, LW_SERVOR_MAX, LW_SERVOR_MIN, LW_SERVOL_MAX, LW_SERVOL_MIN, LW_SERVOR_CON)


out = LW_SERVOR_REV;
end
